simulink model "Controllo_Traccia_uniciclo"  (R2021b)
settings: Solver=ode1be  StartTime=0.0  StopTime=2  FixedStep=1e-3  RelTol=1e-3
values from neighbouring files (symbols this model uses):
  kth = 20    [init.m]
  q0 = [1; 5; pi/2]    [init.m]
  v0 = 10    [init.m]
settings Model: Creator=vince  LastModifiedBy=vince

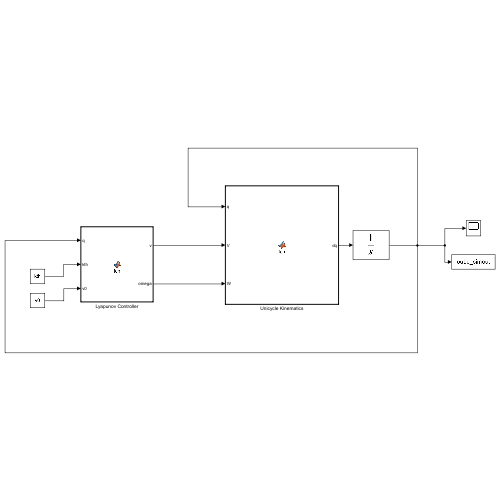
[thumbnail: Simulink's stored preview of the top-level diagram]
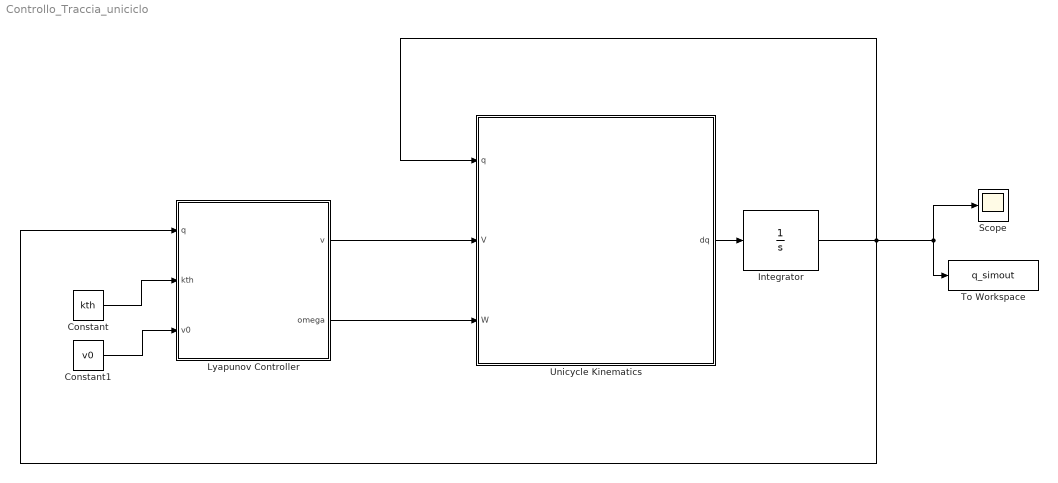
== system Controllo_Traccia_uniciclo ==
  Constant : Constant  Value=kth
  Constant1 : Constant  Value=v0
  Integrator : Integrator  InitialCondition=q0
  Lyapunov Controller : MATLAB Function  TreatAsAtomicUnit=on
  Scope : Scope
  To Workspace : ToWorkspace  VariableName=q_simout  SaveFormat=Timeseries  SampleTime=-1
  Unicycle Kinematics : MATLAB Function  TreatAsAtomicUnit=on
  wires:
  Integrator/1 -> Unicycle Kinematics/1(q), Lyapunov Controller/1(q), Scope/1, To Workspace/1
  Lyapunov Controller/1(v) -> Unicycle Kinematics/2(V)
  Unicycle Kinematics/1(dq) -> Integrator/1
  Lyapunov Controller/2(omega) -> Unicycle Kinematics/3(W)
  Constant/1 -> Lyapunov Controller/2(kth)
  Constant1/1 -> Lyapunov Controller/3(v0)

== matlab function Controllo_Traccia_uniciclo/Lyapunov Controller ==
  data: q input; v output; kth input; omega output; v0 input
function [v, omega] = fcn(q, kth, v0)

y = q(2); th = q(3);


% control
v = v0;

% se x tende a 0 allora sen(x)/x = 1
if th <= 0.0001
    omega = -y*v - kth*th;
else
    omega = -y*(sin(th)/th)*v - kth*th;
end

== matlab function Controllo_Traccia_uniciclo/Unicycle Kinematics ==
  data: q input; dq output; V input; W input
function dq = fcn(q, V, W)

x = q(1); y = q(2); th = q(3);

dx = V * cos(th);
dy = V * sin(th);
dth = W;

dq = [dx; dy; dth];
